simulink model "C_PI_test"  (R2021a)
settings: Solver=VariableStepAuto  StartTime=0.0  StopTime=0.3  RelTol=1e-3
model workspace (MAT data in the model file):
  Kp = 1
  T = 0.001
  T1 = 0.01
  T2 = 0.1
  Tn = 0.1
  v = 4
libraries: Regler x6
settings Model: OrderedModelArguments=off  Creator=Manoli  LastModifiedBy=Manoli

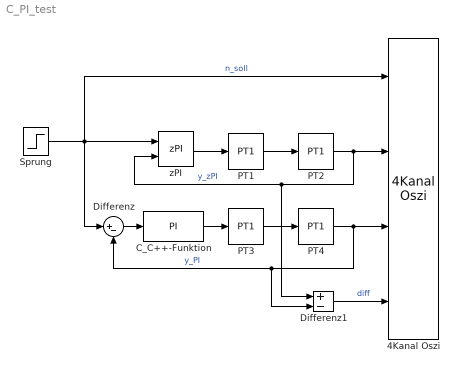
== system C_PI_test ==
  4Kanal Oszi : Regler/4Kanal Oszi  N=20000  k=[1 1 1 1]  y=[-5 5]  tmax=1
  C_C++-Funktion : S-Function  FunctionName=PI  Parameters=T  SFunctionDeploymentMode=off  EnableBusSupport=off
  Differenz : Sum  Inputs=|+-  InputSameDT=on  SaturateOnIntegerOverflow=on  OutDataTypeStr=Inherit: Same as first input
  Differenz1 : Sum  Inputs=+-  InputSameDT=on  SaturateOnIntegerOverflow=on  OutDataTypeStr=Inherit: Same as first input
  PT1 : Regler/PT1  k=v  T1=T1
  PT2 : Regler/PT1  k=v  T1=T2
  PT3 : Regler/PT1  k=v  T1=T1
  PT4 : Regler/PT1  k=v  T1=T2
  Sprung : Step  Time=0.000001  SampleTime=0
  zPI : Regler/zPI  kp=Kp  Tn=Tn  T=T
  wires:
  PT1/1 -> PT2/1
  Sprung/1 -> Differenz/1, 4Kanal Oszi/1, zPI/1  "n_soll"
  zPI/1 -> PT1/1
  PT3/1 -> PT4/1
  PT2/1 -> Differenz1/1, zPI/2, 4Kanal Oszi/2  "y_zPI"
  C_C++-Funktion/1 -> PT3/1
  PT4/1 -> Differenz1/2, Differenz/2, 4Kanal Oszi/3  "y_PI"
  Differenz/1 -> C_C++-Funktion/1
  Differenz1/1 -> 4Kanal Oszi/4  "diff"
